simulink model "simulink_practica5"  (R2025b)
settings: Solver=VariableStepAuto  StartTime=0.0  StopTime=10.0  RelTol=1e-3

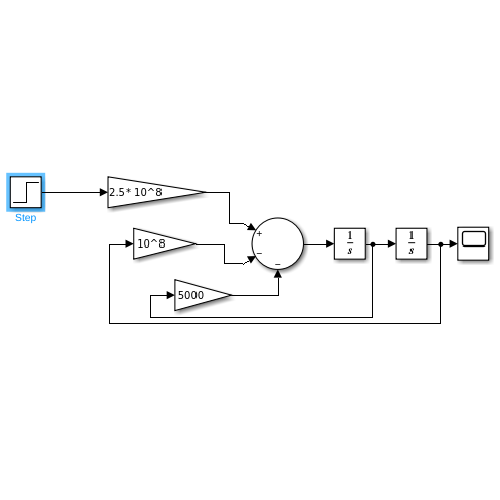
[thumbnail: Simulink's stored preview of the top-level diagram]
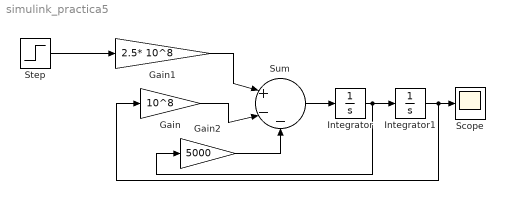
== system simulink_practica5 ==
  Gain : Gain  Gain=10^8
  Gain1 : Gain  Gain=2.5* 10^8
  Gain2 : Gain  Gain=5000
  Integrator : Integrator
  Integrator1 : Integrator
  Scope : Scope
      settings: ActiveDisplayYMinimum=2.4950781633934156  ActiveDisplayYMaximum=2.5050484454396362
  Step : Step  SampleTime=0
  Sum : Sum  Inputs=|+--
  wires:
  Gain1/1 -> Sum/1
  Gain/1 -> Sum/2
  Gain2/1 -> Sum/3
  Step/1 -> Gain1/1
  Sum/1 -> Integrator/1
  Integrator/1 -> Gain2/1, Integrator1/1
  Integrator1/1 -> Gain/1, Scope/1
